simulink model "HydraLeg"  (R2014b)
settings: Solver=ode3  StartTime=0.0  StopTime=inf  FixedStep=tModel  RelTol=1e-3
undefined symbols (not defined in the file or in its folder): Circum, gcbh, lever, lightThreshold, rmidispblock, tModel
libraries: legoev3lib x14, simulink x5, EV3Fcns x4
settings Model: DataDictionary=HydraLeg.sldd  ExtModeTrigDuration=2  Creator=menkh  LastModifiedBy=menkh
settings OptimizationCC: OptimizeModelRefInitCode=on  LifeSpan=1
settings DebuggingCC: UnderspecifiedInitializationDetection=Classic  MergeDetectMultiDrivingBlocksExec=none  SolverPrmCheckMsg=none
settings HardwareCC: ProdLargestAtomicInteger=Long  ProdLargestAtomicFloat=Float  ProdEndianess=LittleEndian  ProdHWDeviceType=ARM Compatible->ARM 9
settings RTWCC: SystemTargetFile=realtime.tlc  GenerateMakefile=off  TemplateMakefile=realtime.tmf  Description=Run on Target Hardware  RTWVerbose=off  ProcessScript=realtime_make_rtw_hook
settings STFCustomTargetCC: TargetLibSuffix=.a  GenerateSampleERTMain=on  CombineSignalStateStructs=on  ERTCustomFileBanners=on  SupportNonInlinedSFcns=off  SupportVariableSizeSignals=on  MATLABClassNameForMDSCustomization=Simulink.SoftwareTarget.ERTCustomization  GRTInterface=off  SystemTargetFile=realtime.tlc
settings ERTTargetCC: GenerateSampleERTMain=on  ParMdlRefBuildCompliant=off  CompOptLevelCompliant=off  ConcurrentExecutionCompliant=off  CombineOutputUpdateFcns=off  CombineSignalStateStructs=on  ERTFirstTimeCompliant=off  SupportContinuousTime=on  SupportVariableSizeSignals=on  ModelStepFunctionPrototypeControlCompliant=off  CPPClassGenCompliant=off  InlinedParameterPlacement=NonHierarchical  ERTSrcFileBannerTemplate=realtime_code_template.cgt  ERTHdrFileBannerTemplate=realtime_code_template.cgt  ERTDataSrcFileTemplate=realtime_code_template.cgt  ERTDataHdrFileTemplate=realtime_code_template.cgt  ERTCustomFileTemplate=realtime_file_process.tlc

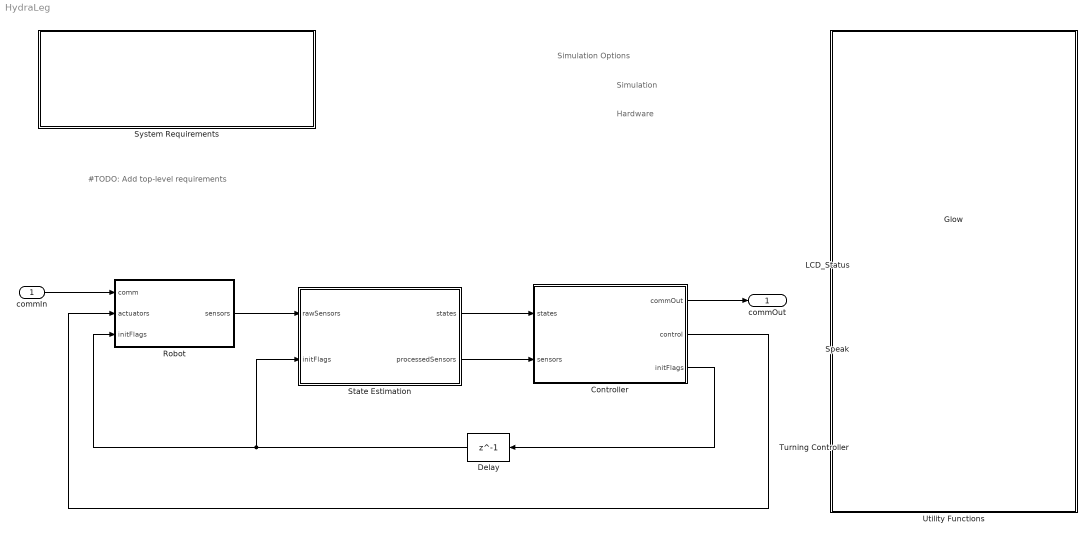
== system HydraLeg ==
  note: #TODO:
      | Add top-level requirements
  note: Simulation Options
  note: Simulation
  note: Hardware
  commIn : Inport  OutDataTypeStr=Enum: Comm
  Controller : Stateflow chart  TreatAsAtomicUnit=on
  Delay : Delay  DelayLength=1  SampleTime=tModel
      settings: AttributesFormatString=Removes algebraic loop
  Glow : EV3Fcns/Glow
  LCD_Status : EV3Fcns/LCD_Status
  Robot : Subsystem  Variant=on  VariantControl=Variant1  OverrideUsingVariant=HardwareVar
  Speak : EV3Fcns/Speak
  State Estimation : Subsystem
  System Requirements : Subsystem  LoadFcn=rmidispblock('load',gcbh)  mask(System Requirements){id=SystemReq, title=System Requirements}
      mask prompts: title "Block Title"
      mask help: Lists the requirements for the current model.
      mask init:
      | id = 'SystemReq';
      | [w,h] = rmidispblock('display',gcbh);
      settings: CopyFcn=rmidispblock('create',gcbh)  DeleteFcn=rmidispblock('delete',gcbh)  ModelCloseFcn=rmidispblock('close',gcbh)  PreSaveFcn=rmidispblock('close',gcbh)  PostSaveFcn=rmidispblock('open',gcbh)  OpenFcn=rmidispblock('open',gcbh)  MoveFcn=rmidispblock('move',gcbh)
      mask Help: helpview(fullfile(docroot,'toolbox','slvnv','slvnv.map'),'systemrequirements')
      mask Display:
      | text(326/2,113-4,rmidispblock('title',gcbh),'horizontalAlignment','center','verticalAlignment','top')
      | text(w/2,h/2,'<No Requirements in System>','horizontalAlignment','center','verticalAlignment','top')
  Turning Controller : EV3Fcns/Turning Controller
      link override Saturation: UpperLimit=2  LowerLimit=-2
  Utility Functions : Subsystem
  commOut : Outport  OutDataTypeStr=Enum: Comm
  wires:
  State Estimation/2(processedSensors) -> Controller/2(sensors)
  Robot/1(sensors) -> State Estimation/1(rawSensors)
  Controller/3(initFlags) -> Delay/1
  State Estimation/1(states) -> Controller/1(states)
  Delay/1 -> Robot/3(initFlags), State Estimation/2(initFlags)
  Controller/2(control) -> Robot/2(actuators)
  Controller/1(commOut) -> commOut/1
  commIn/1 -> Robot/1(comm)

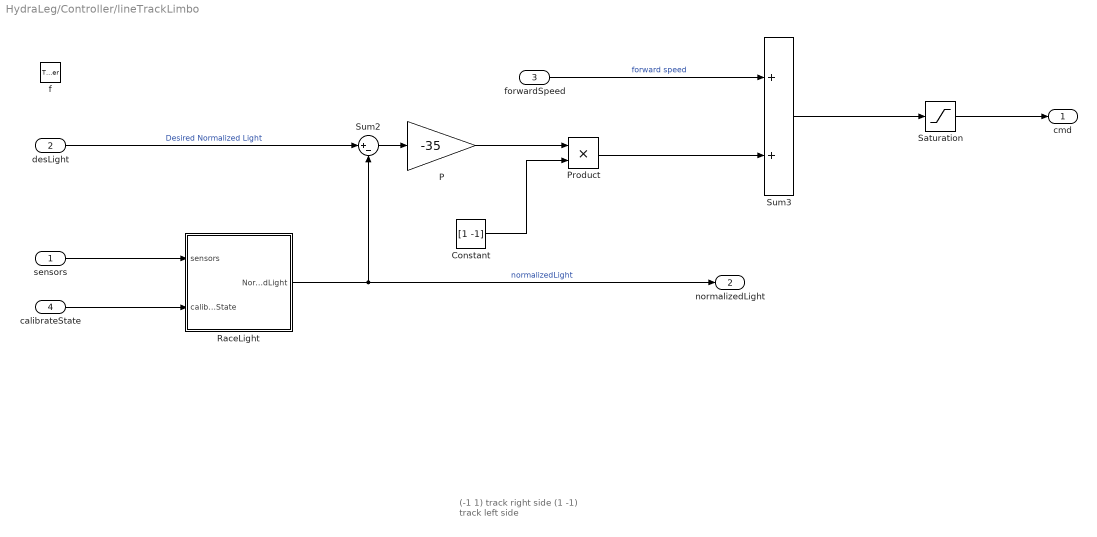
== system HydraLeg/Controller/lineTrackLimbo ==
  note: (-1 1)  track right side
      | (1 -1)  track left side
  sensors : Inport  OutDataTypeStr=single  PortDimensions=1  LockScale=on
  desLight : Inport  Port=2  OutDataTypeStr=single  PortDimensions=1
  forwardSpeed : Inport  Port=3  OutDataTypeStr=single  PortDimensions=2
  calibrateState : Inport  Port=4  OutDataTypeStr=boolean  PortDimensions=1  LockScale=on
  f : TriggerPort  TriggerType=function-call
      settings: CopyFcn=Stateflow.SLINSF.SimulinkMan.removeBlockPreDeleteFcn  PreDeleteFcn=Stateflow.SLINSF.SimulinkMan.unsafePredeleteFcn
  Constant : Constant  Value=[1 -1]  OutDataTypeStr=single  SampleTime=-1
  P : Gain  Gain=-35
  Product : Product
  RaceLight : Subsystem
  Saturation : Saturate  UpperLimit=100  LowerLimit=-100  OutDataTypeStr=single
  Sum2 : Sum  Inputs=|+-
  Sum3 : Sum
  cmd : Outport  OutDataTypeStr=single  PortDimensions=2
  normalizedLight : Outport  Port=2  OutDataTypeStr=single  PortDimensions=1
  wires:
  P/1 -> Product/1
  forwardSpeed/1 -> Sum3/1  "forward speed"
  Saturation/1 -> cmd/1
  Sum2/1 -> P/1
  desLight/1 -> Sum2/1  "Desired Normalized Light"
  sensors/1 -> RaceLight/1(sensors)
  RaceLight/1(NormalizedLight) -> normalizedLight/1, Sum2/2  "normalizedLight"
  Constant/1 -> Product/2
  Sum3/1 -> Saturation/1
  Product/1 -> Sum3/2
  calibrateState/1 -> RaceLight/2(calibrateState)

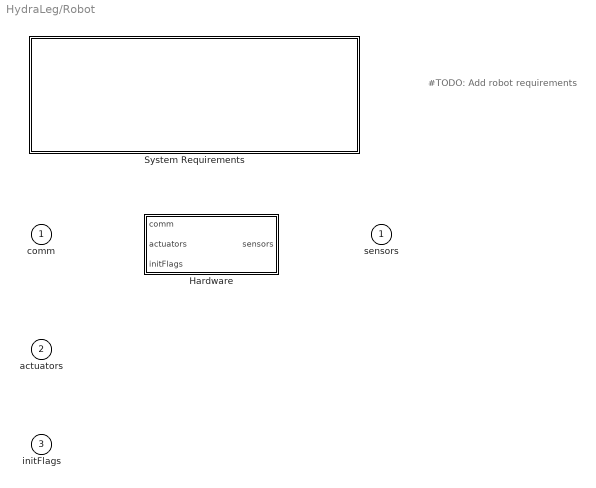
== system HydraLeg/Robot ==
  note: #TODO:
      | Add robot requirements
  comm : Inport  OutDataTypeStr=Enum: Comm
  actuators : Inport  Port=2  OutDataTypeStr=Bus: ControlBus
  initFlags : Inport  Port=3  OutDataTypeStr=Bus: InitBus
  Hardware : Subsystem  VariantControl=HardwareVar
  System Requirements : Subsystem  LoadFcn=rmidispblock('load',gcbh)  VariantControl=Variant  mask(System Requirements){id=SystemReq, title=System Requirements}
      mask prompts: title "Block Title"
      mask help: Lists the requirements for the current model.
      mask init:
      | id = 'SystemReq';
      | [w,h] = rmidispblock('display',gcbh);
      settings: CopyFcn=rmidispblock('create',gcbh)  DeleteFcn=rmidispblock('delete',gcbh)  ModelCloseFcn=rmidispblock('close',gcbh)  PreSaveFcn=rmidispblock('close',gcbh)  PostSaveFcn=rmidispblock('open',gcbh)  OpenFcn=rmidispblock('open',gcbh)  MoveFcn=rmidispblock('move',gcbh)
      mask Help: helpview(fullfile(docroot,'toolbox','slvnv','slvnv.map'),'systemrequirements')
      mask Display:
      | text(326/2,113-4,rmidispblock('title',gcbh),'horizontalAlignment','center','verticalAlignment','top')
      | text(w/2,h/2,'<No Requirements in System>','horizontalAlignment','center','verticalAlignment','top')
  sensors : Outport  OutDataTypeStr=Bus: Sensors_Bus

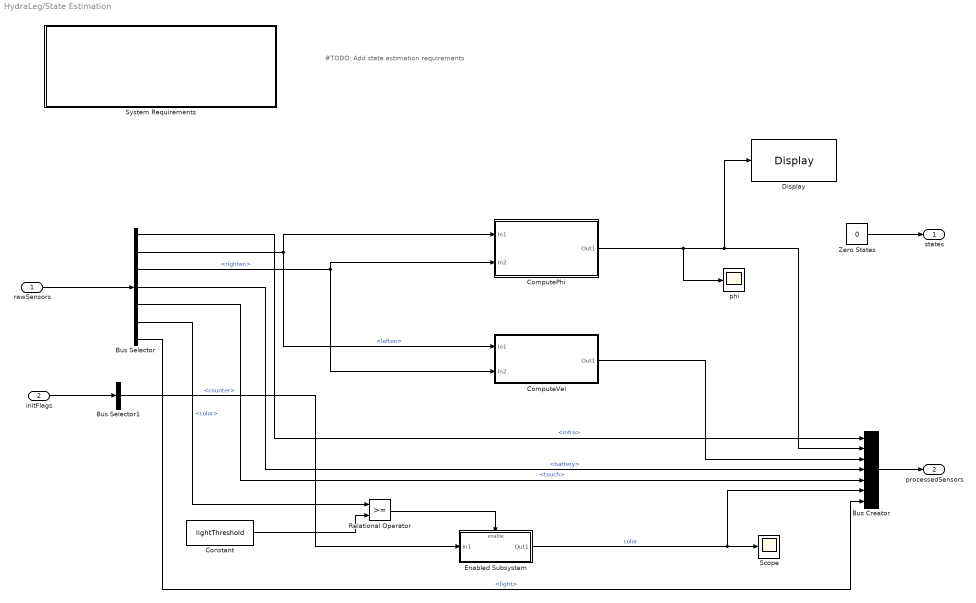
== system HydraLeg/State Estimation ==
  note: #TODO:
      | Add state estimation requirements
  rawSensors : Inport  OutDataTypeStr=Bus: Sensors_Bus
  initFlags : Inport  Port=2  OutDataTypeStr=Bus: InitBus
  Bus Creator : BusCreator  Inputs=7
  Bus Selector : BusSelector  OutputSignals=infra,leften,righten,battery,touch,color,light
  Bus Selector1 : BusSelector  OutputSignals=counter
  ComputePhi : Subsystem
  ComputeVel : Subsystem
  Constant : Constant  Value=lightThreshold
  Display : legoev3lib/Display  slcdStr=phi  slcdLine=3  slcdFormat=Decimal
  Enabled Subsystem : Subsystem  TreatAsAtomicUnit=on
  Relational Operator : RelationalOperator  OutDataTypeStr=boolean
  Scope : Scope
      settings: YMin=43  YMax=45  SaveName=ScopeData2
  System Requirements : Subsystem  LoadFcn=rmidispblock('load',gcbh)  mask(System Requirements){id=SystemReq, title=System Requirements}
      mask prompts: title "Block Title"
      mask help: Lists the requirements for the current model.
      mask init:
      | id = 'SystemReq';
      | [w,h] = rmidispblock('display',gcbh);
      settings: CopyFcn=rmidispblock('create',gcbh)  DeleteFcn=rmidispblock('delete',gcbh)  ModelCloseFcn=rmidispblock('close',gcbh)  PreSaveFcn=rmidispblock('close',gcbh)  PostSaveFcn=rmidispblock('open',gcbh)  OpenFcn=rmidispblock('open',gcbh)  MoveFcn=rmidispblock('move',gcbh)
      mask Help: helpview(fullfile(docroot,'toolbox','slvnv','slvnv.map'),'systemrequirements')
      mask Display:
      | text(326/2,113-4,rmidispblock('title',gcbh),'horizontalAlignment','center','verticalAlignment','top')
      | text(w/2,h/2,'<No Requirements in System>','horizontalAlignment','center','verticalAlignment','top')
  Zero States : Constant  Value=0  OutDataTypeStr=Bus: States_Bus  SampleTime=tModel
  phi : Scope
      settings: YMin=-1  YMax=1  SaveName=ScopeData3
  states : Outport  OutDataTypeStr=Bus: States_Bus
  processedSensors : Outport  Port=2  OutDataTypeStr=Bus: PSensors_Bus
  wires:
  initFlags/1 -> Bus Selector1/1
  Zero States/1 -> states/1
  rawSensors/1 -> Bus Selector/1
  Bus Selector/5 -> Bus Creator/5  "<touch>"
  Bus Selector/3 -> ComputeVel/2(In2), ComputePhi/2(In2)  "<righten>"
  Bus Selector/2 -> ComputePhi/1(In1), ComputeVel/1(In1)  "<leften>"
  Bus Selector/4 -> Bus Creator/4  "<battery>"
  Bus Creator/1 -> processedSensors/1
  ComputePhi/1(Out1) -> phi/1, Display/1, Bus Creator/2
  ComputeVel/1(Out1) -> Bus Creator/3
  Bus Selector/1 -> Bus Creator/1  "<infra>"
  Bus Selector/6 -> Relational Operator/1  "<color>"
  Relational Operator/1 -> Enabled Subsystem/Enable
  Constant/1 -> Relational Operator/2
  Enabled Subsystem/1(Out1) -> Scope/1, Bus Creator/6  "color"
  Bus Selector1/1 -> Enabled Subsystem/1(In1)  "<counter>"
  Bus Selector/7 -> Bus Creator/7  "<light>"

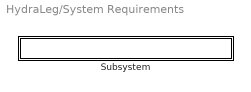
== system HydraLeg/System Requirements ==
  Subsystem : Subsystem  mask{label=0, index=1}
      mask init:
      | label = rmidispblock('label',index);
      settings: OpenFcn=rmidispblock('openReq',gcbh);
      mask Display: text(0,0,label,'horizontalAlignment','left','verticalAlignment','bottom')

== system HydraLeg/Utility Functions ==

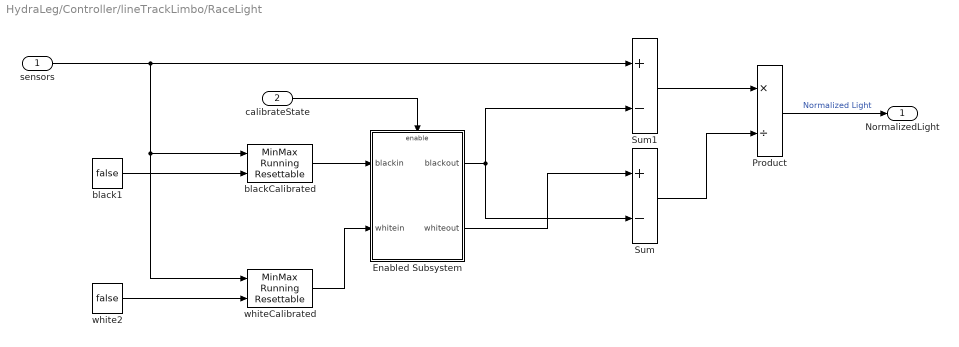
== system HydraLeg/Controller/lineTrackLimbo/RaceLight ==
  sensors : Inport  OutDataTypeStr=single  PortDimensions=1  LockScale=on
  calibrateState : Inport  Port=2  OutDataTypeStr=boolean  PortDimensions=1  LockScale=on
  Enabled Subsystem : Subsystem  TreatAsAtomicUnit=on
  Product : Product  Inputs=*/
  Sum : Sum  Inputs=+-
  Sum1 : Sum  Inputs=+-
  black1 : Constant  Value=false  OutDataTypeStr=boolean  SampleTime=-1
  "blackCalibrated " : simulink/Math Operations/MinMax Running Resettable  Function=min  vinit=10
  white2 : Constant  Value=false  OutDataTypeStr=boolean  SampleTime=-1
  whiteCalibrated : simulink/Math Operations/MinMax Running Resettable  Function=max  vinit=90
  NormalizedLight : Outport
  wires:
  Sum1/1 -> Product/1
  Sum/1 -> Product/2
  whiteCalibrated/1 -> Enabled Subsystem/2(whitein)
  sensors/1 -> Sum1/1, "blackCalibrated "/1, whiteCalibrated/1
  Product/1 -> NormalizedLight/1  "Normalized Light"
  black1/1 -> "blackCalibrated "/2
  white2/1 -> whiteCalibrated/2
  "blackCalibrated "/1 -> Enabled Subsystem/1(blackin)
  Enabled Subsystem/1(blackout) -> Sum1/2, Sum/2
  Enabled Subsystem/2(whiteout) -> Sum/1
  calibrateState/1 -> Enabled Subsystem/Enable

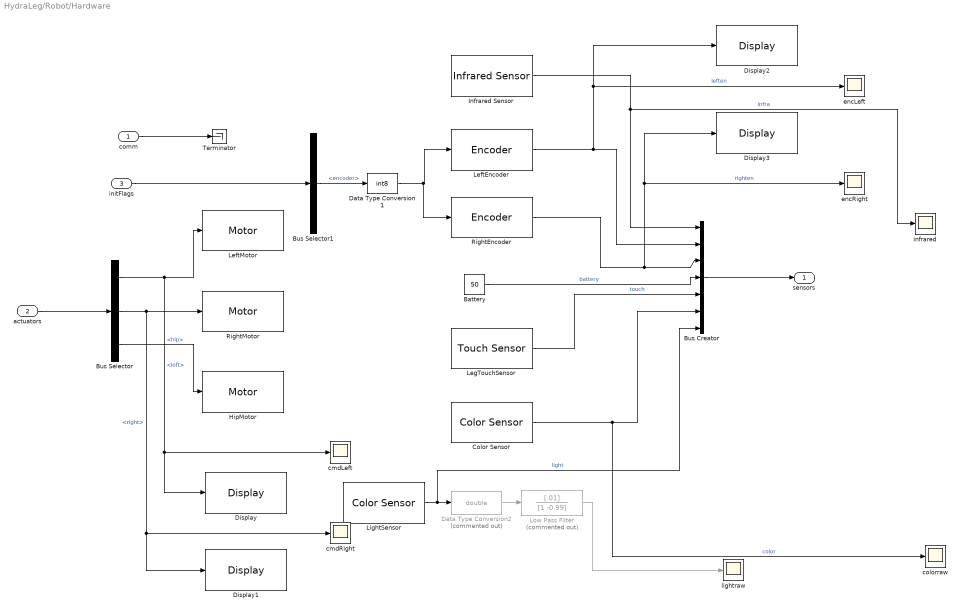
== system HydraLeg/Robot/Hardware ==
  comm : Inport
  actuators : Inport  Port=2
  initFlags : Inport  Port=3
  Battery : Constant  Value=50  OutDataTypeStr=uint8  SampleTime=tModel
  Bus Creator : BusCreator  Inputs=7  OutDataTypeStr=Bus: Sensors_Bus
  Bus Selector : BusSelector  OutputSignals=left,right,hip
  Bus Selector1 : BusSelector  OutputSignals=encoder
  Color Sensor : legoev3lib/Color Sensor  portNumber=4  mode=Ambient light intensity  sampleTime=tModel
  Data Type Conversion1 : DataTypeConversion  OutDataTypeStr=int8
  Data Type Conversion2 : DataTypeConversion  Commented=on  OutDataTypeStr=double
  Display : legoev3lib/Display  slcdStr=Left  slcdLine=1  slcdFormat=Decimal
  Display1 : legoev3lib/Display  slcdStr=Right  slcdLine=2  slcdFormat=Decimal
  Display2 : legoev3lib/Display  slcdStr=LeftEn  slcdLine=4  slcdFormat=Decimal
  Display3 : legoev3lib/Display  slcdStr=RightEn  slcdLine=5  slcdFormat=Decimal
  HipMotor : legoev3lib/Motor  sportNumber=D  sstopAction=Brake
  Infrared Sensor : legoev3lib/Infrared Sensor  portNumber=2  channelNumber=1  sampleTime=tModel
  LeftEncoder : legoev3lib/Encoder  portNumber=B  opMode=Reset by external signal  sampleTime=tModel
  LeftMotor : legoev3lib/Motor  sportNumber=B  sstopAction=Brake
  LegTouchSensor : legoev3lib/Touch Sensor  portNumber=1  sampleTime=tModel
  LightSensor : legoev3lib/Color Sensor  portNumber=3  mode=Reflected light intensity  sampleTime=tModel
  Low Pass Filter : DiscreteFilter  Commented=on  Numerator=[.01]  Denominator=[1 -0.99]
  RightEncoder : legoev3lib/Encoder  portNumber=A  opMode=Reset by external signal  sampleTime=tModel
  RightMotor : legoev3lib/Motor  sportNumber=A  sstopAction=Brake
  Terminator : Terminator
  cmdLeft : Scope
      settings: YMin=7  YMax=8  SaveName=ScopeData4
  cmdRight : Scope
      settings: YMin=7  YMax=8  SaveName=ScopeData5
  colorraw : Scope
      settings: YMin=0  YMax=1
  encLeft : Scope
      settings: YMin=-1  YMax=1  SaveName=ScopeData6
  encRight : Scope
      settings: TimeRange=10  YMin=7  YMax=8  SaveName=ScopeData7
  infrared : Scope
      settings: TimeRange=10  YMin=0  YMax=9  SaveName=ScopeData8
  lightraw : Scope
      settings: YMin=9.75  YMax=10.15
  sensors : Outport  OutDataTypeStr=Bus: Sensors_Bus
  wires:
  comm/1 -> Terminator/1
  Bus Selector/1 -> cmdLeft/1, Display/1, LeftMotor/1  "<left>"
  actuators/1 -> Bus Selector/1
  Bus Selector/2 -> Display1/1, cmdRight/1, RightMotor/1  "<right>"
  Bus Selector/3 -> HipMotor/1  "<hip>"
  LegTouchSensor/1 -> Bus Creator/5  "touch"
  Battery/1 -> Bus Creator/4  "battery"
  Bus Creator/1 -> sensors/1
  RightEncoder/1 -> encRight/1, Display3/1, Bus Creator/3  "righten"
  LeftEncoder/1 -> encLeft/1, Display2/1, Bus Creator/2  "leften"
  Infrared Sensor/1 -> infrared/1, Bus Creator/1  "infra"
  initFlags/1 -> Bus Selector1/1
  Bus Selector1/1 -> Data Type Conversion1/1  "<encoder>"
  Data Type Conversion1/1 -> RightEncoder/1, LeftEncoder/1
  Color Sensor/1 -> colorraw/1, Bus Creator/6  "color"
  LightSensor/1 -> Bus Creator/7, Data Type Conversion2/1  "light"
  Low Pass Filter/1 -> lightraw/1
  Data Type Conversion2/1 -> Low Pass Filter/1

== system HydraLeg/Robot/System Requirements ==
  Subsystem : Subsystem  mask{label=0, index=1}
      mask init:
      | label = rmidispblock('label',index);
      settings: OpenFcn=rmidispblock('openReq',gcbh);
      mask Display: text(0,0,label,'horizontalAlignment','left','verticalAlignment','bottom')

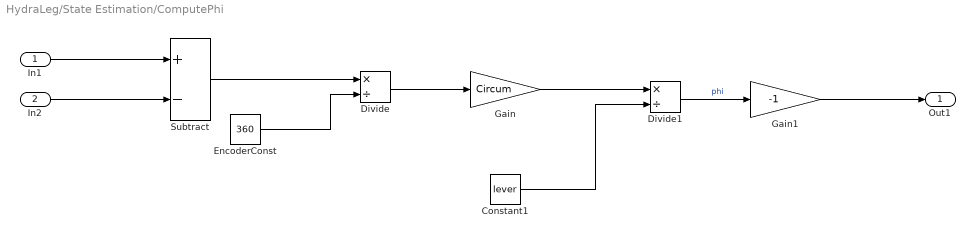
== system HydraLeg/State Estimation/ComputePhi ==
  In1 : Inport
  In2 : Inport  Port=2
  Constant1 : Constant  Value=lever  OutDataTypeStr=single  SampleTime=tModel
  Divide : Product  Inputs=*/  OutDataTypeStr=single
  Divide1 : Product  Inputs=*/  OutDataTypeStr=single
  EncoderConst : Constant  Value=360  OutDataTypeStr=int32  SampleTime=tModel
  Gain : Gain  Gain=Circum  OutDataTypeStr=single
  Gain1 : Gain  Gain=-1  OutDataTypeStr=single
  Subtract : Sum  Inputs=+-
  Out1 : Outport
  wires:
  Divide1/1 -> Gain1/1  "phi"
  Gain/1 -> Divide1/1
  Divide/1 -> Gain/1
  Subtract/1 -> Divide/1
  Constant1/1 -> Divide1/2
  EncoderConst/1 -> Divide/2
  In1/1 -> Subtract/1
  In2/1 -> Subtract/2
  Gain1/1 -> Out1/1

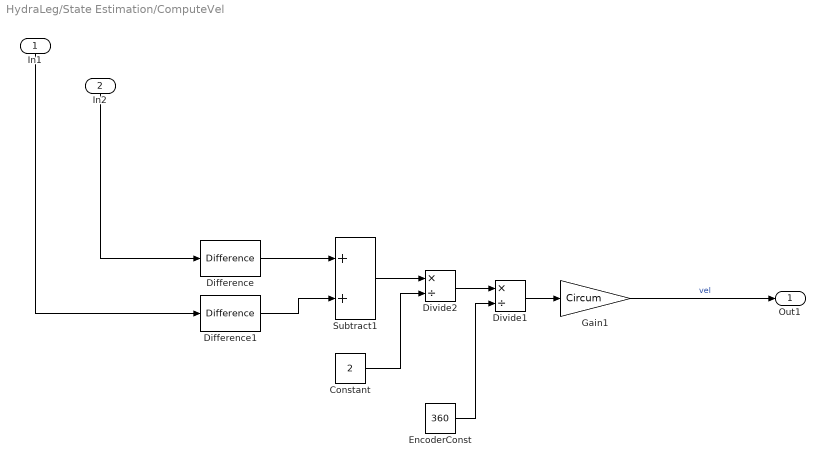
== system HydraLeg/State Estimation/ComputeVel ==
  In1 : Inport
  In2 : Inport  Port=2
  Constant : Constant  Value=2  OutDataTypeStr=uint8  SampleTime=tModel
  Difference : simulink/Discrete/Difference  ICPrevInput=0.0  InputProcessing=Inherited  OutMin=[]  OutMax=[]  OutDataTypeStr=single  OutputDataTypeScalingMode=single  OutDataType=fixdt(1, 16)  OutScaling=2^-10  DoSatur=off
  Difference1 : simulink/Discrete/Difference  ICPrevInput=0.0  InputProcessing=Inherited  OutMin=[]  OutMax=[]  OutDataTypeStr=single  OutputDataTypeScalingMode=single  OutDataType=fixdt(1, 16)  OutScaling=2^-10  DoSatur=off
  Divide1 : Product  Inputs=*/  OutDataTypeStr=single
  Divide2 : Product  Inputs=*/  OutDataTypeStr=single
  EncoderConst : Constant  Value=360  OutDataTypeStr=single  SampleTime=tModel
  Gain1 : Gain  Gain=Circum  OutDataTypeStr=single
  Subtract1 : Sum
  Out1 : Outport
  wires:
  Gain1/1 -> Out1/1  "vel"
  Subtract1/1 -> Divide2/1
  Constant/1 -> Divide2/2
  Difference/1 -> Subtract1/1
  In2/1 -> Difference/1
  Difference1/1 -> Subtract1/2
  In1/1 -> Difference1/1
  Divide2/1 -> Divide1/1
  Divide1/1 -> Gain1/1
  EncoderConst/1 -> Divide1/2

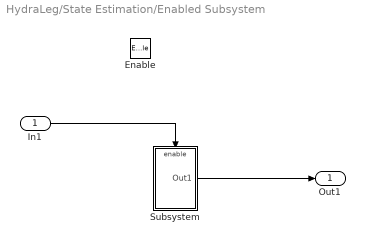
== system HydraLeg/State Estimation/Enabled Subsystem ==
  In1 : Inport
  Enable : EnablePort
  Subsystem : Subsystem
  Out1 : Outport
  wires:
  Subsystem/1(Out1) -> Out1/1
  In1/1 -> Subsystem/Enable

== system HydraLeg/State Estimation/System Requirements ==
  Subsystem : Subsystem  mask{label=0, index=1}
      mask init:
      | label = rmidispblock('label',index);
      settings: OpenFcn=rmidispblock('openReq',gcbh);
      mask Display: text(0,0,label,'horizontalAlignment','left','verticalAlignment','bottom')

== system HydraLeg/System Requirements/Subsystem ==

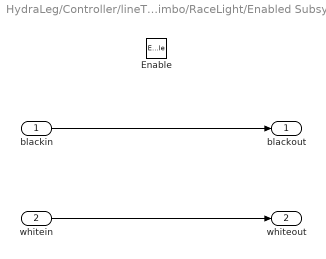
== system HydraLeg/Controller/lineTrackLimbo/RaceLight/Enabled Subsystem ==
  blackin : Inport
  whitein : Inport  Port=2
  Enable : EnablePort
  blackout : Outport
  whiteout : Outport  Port=2
  wires:
  blackin/1 -> blackout/1
  whitein/1 -> whiteout/1

== system HydraLeg/Robot/System Requirements/Subsystem ==

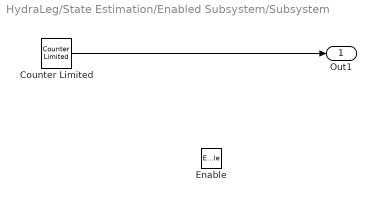
== system HydraLeg/State Estimation/Enabled Subsystem/Subsystem ==
  Enable : EnablePort  StatesWhenEnabling=reset
  Counter Limited : simulink/Sources/Counter Limited  uplimit=100  tsamp=-1
  Out1 : Outport
  wires:
  Counter Limited/1 -> Out1/1

== system HydraLeg/State Estimation/System Requirements/Subsystem ==

== stateflow chart HydraLeg/Controller ==
  note: #TODO
      | Add requirements to Stateflow objects
      | by right-clicking and selecting the
      | Requirements Traceability option.
  state initBuses [function]
    (default) -> (junction 186) : % Control bus
        | {
        | control.left = int8(0);
        | control.right = int8(0);
        | control.hip = int8(0);
        | }
    (junction 186) -> (junction 187) : % Initialization flags
        | {
        | initFlags.encoder = true;
        | initFlags.gyro = true;
        | initFlags.counter = true;
        | phicum = single(0);
        | }
  state NOPState
    en:
    n = single(1);
    initBuses();
    Speak(2);
    commOut = Comm.NONE;
    phicum = single(0);
    initFlags.counter = false;
    normalizedLight = single(0.5);
    du:
    Glow(1);
  state LegAction
    en:
    n = single(0);
    initFlags.encoder = false;
    initFlags.gyro = false;
    initFlags.counter = true;
    du:
    Glow(4);
    state initialPosition1
    state CalibrateLight
      en, du:
      StatusLCD(10);
      Glow(2);
      lineTrackLimbo(single(sensors.light),single(0.5), single([50; 50]), true);
      state rotateright
        en, du:
        move(-45, 0, 20);
      state rotateleft
        en, du:
        move(45, 0, 20);
      state initialPosition1
        en:
        stop();
      state initialPosition2
        en:
        stop();
      state initialPosition
        en, du:
        move(0, 0, 20);
      LegAction.CalibrateLight.initialPosition1 -> rotateright : after(1, sec)
      rotateright -> initialPosition2 : [sensors.phi <= -45]
      (default) -> rotateleft
      rotateleft -> LegAction.CalibrateLight.initialPosition1 : [sensors.phi >= 45]
      initialPosition2 -> initialPosition : after(1, sec)
    state WaitForLight
      en,du:
      StatusLCD(400);
      Glow(1);
    state Turn
      en,du:
      StatusLCD(300);
      move(45, 0, 20);
      Glow(4);
    state Turn1
      en:
      StatusLCD(300);
      Glow(4); %blink green
    state Wait1
      en:
      stop();
      Glow(4);
    state WarZoneStop
      en,du:
      StatusLCD(400);
      Glow(3);
      stop();
      Speak(50);
    state LineTrack
      en, du:
      StatusLCD(500);
      Glow(6); %blink orange
      linetrack(30);
    state Wait2
      en, du:
      stop();
      Glow(4);
      Speak(50);
    state WZBackward
      en,du:
      StatusLCD(400);
      Glow(2);
      move(0, -40, 0);
    state Turn2
      en,du:
      move(0, 0, 20);
      Glow(4);
      normalizedLight = getNormalizedLight();
    state WZForward
      en,du:
      StatusLCD(400);
      Glow(2);
      move(0, 40, 0);
    state Rotate360
      en:
      stop();
      du:
      move(495,0,20);
      Glow(5);
    state WZStop
      en, du:
      stop();
      Glow(2);
      Speak(50);
    state WZStop1
      en, du:
      stop();
      Glow(2);
      Speak(50);
    state RotateToNXT
      en,du:
      StatusLCD(400);
      Glow(5);
      control.left = int8(40);
      control.right = int8(-40);
    state RotateToNXT2
      en,du:
      Glow(5);
      control.left = int8(30);
      control.right = int8(-30);
      normalizedLight = getNormalizedLight();
    state WZBackward10
      en,du:
      StatusLCD(400);
      Glow(2);
      move(0, -40, 0);
    state Stop
      en,du:
      stop();
      Glow(5);
    state LineTrack2
      en, du:
      StatusLCD(500);
      Glow(5);
      linetrack(20);
      Speak(50);
    state Rotate
      en:
      stop();
      du:
      move(300,0,20);
      Glow(5);
      Speak(50);
    state AttackNXT
      en,du:
      move(0, 50, 0);
      Glow(5);
    LegAction.initialPosition1 -> CalibrateLight : after(1, sec)
    (default) -> LegAction.initialPosition1
    Turn1 -> Turn : after(3,sec)
    WaitForLight -> Turn1 : [sensors.color>= 100]
    Turn -> Wait1 : [sensors.phi >= 45]
    LineTrack -> WarZoneStop : after(34,sec)
    Wait1 -> Turn2 : after(15, sec)
    Wait2 -> LineTrack : after(2, sec)
    WarZoneStop -> WZBackward : after(2,sec)
    Turn2 -> Wait2 : [sensors.phi <= 0 || normalizedLight <= 0.5]
    WZBackward -> WZStop : after(2, sec)
    WZForward -> Rotate360 [order 2] : after(2, sec)
    WZForward -> WZStop1 [order 1] : after(2, sec)
    Rotate360 -> WZStop1 : after(2, sec)
    WZStop -> WZForward : after(2, sec)
    WZStop1 -> WZBackward10 : after(2, sec)
    RotateToNXT -> RotateToNXT2 : after(2, sec)
    WZBackward10 -> RotateToNXT : after(2, sec)
    RotateToNXT2 -> LineTrack2 : [normalizedLight <= 0.65 || sensors.phi <= -45]
    Rotate -> Stop : [sensors.phi>=300]
    LineTrack2 -> AttackNXT : after(5,sec)
    AttackNXT -> Rotate : after(2, sec)
  state stop [function]
    (default) -> (junction 279) : % Control bus
        | {
        | control.left = int8(0);
        | control.right = int8(0);
        | }
  state linetrack(V) [function]
    (default) -> (junction 345) : % Control bus
        | {
        | [cmdline, nlight] = lineTrackLimbo(single(sensors.light),single(0.5), single([V; V]), false);
        | control.left = int8(cmdline(1));
        | control.right = int8(cmdline(2));
        | }
  state NOPState2
    en:
    stop();
    n = single(1);
    initBuses();
  state move(phi, V, turngain) [function]
    (default) -> (junction 239) : % Control bus
        | {
        | cmd = TurningCtrl(single(phi),sensors.phi, single(turngain));
        | control.left = int8(cmd(1) + V);
        | control.right = int8(cmd(2) + V);
        | }
  state nlight = getNormalizedLight [function]
    (default) -> (junction 393) : % Control bus
        | {
        | [cmdline, nlight] = lineTrackLimbo(single(sensors.light),single(0.5), single([0; 0]), false);
        | }
  state [cmd,normalizedLight] = lineTrackLimbo(sensors,desLight,forwardSpeed,calibrateState) [function]
  initialPosition -> NOPState2 : [sensors.phi >= 0]
  LegAction -> NOPState : [sensors.infra == 1]
      | {calibdone = true}
  (default) -> NOPState : {calibdone = false}
  NOPState -> LegAction [order 1] : [calibdone == false]
  NOPState -> LegAction [order 2] : [sensors.infra == 3]
  NOPState2 -> WaitForLight
  data: V function_input; phi function_input; V function_input; turngain function_input; nlight function_output; sensors function_input single size=1; desLight function_input single size=1; cmd function_output single size=2; forwardSpeed function_input single size=2; calibrateState function_input boolean size=1; normalizedLight function_output single size=1; commOut output Enum: Comm size=1; control output Bus: ControlBus size=1; states input Bus: States_Bus size=1; sensors input Bus: PSensors_Bus size=1; initFlags output Bus: InitBus size=1; n local; cmd local; soundVal parameter; phicum local single; normalizedLight local single size=1; calibdone local boolean size=1
